simulink model "FSFB_FO_DoublePendulum"  (R2023b)
settings: Solver=VariableStepAuto  StartTime=0.0  StopTime=8  RelTol=1e-3
values from neighbouring files (symbols this model uses):
  A = [0 1 0 0; 9.8 0 -9.8 0; 0 0 0 1; -9.8 0 2.94 0]    [FSFB_FO_MIMO_doublePendulum.m]    (also in FSFB_MIMO_doublePendulum.m; FSFB_MO_MIMO_doublePendulum.m)
  B = [0 0; 1 -2; 0 0; -2 5]    [FSFB_FO_MIMO_doublePendulum.m]    (also in FSFB_MIMO_doublePendulum.m; FSFB_MO_MIMO_doublePendulum.m)
  C = [1 0 0 0; 0 0 1 0]    [FSFB_FO_MIMO_doublePendulum.m]    (also in FSFB_MIMO_doublePendulum.m; FSFB_MO_MIMO_doublePendulum.m)
  C_full = eye(max(size(A)))    [FSFB_FO_MIMO_doublePendulum.m]    (also in FSFB_MO_MIMO_doublePendulum.m)
  K_moore = W_moore/V_moore    [FSFB_FO_MIMO_doublePendulum.m]    (also in FSFB_MIMO_doublePendulum.m; FSFB_MO_MIMO_doublePendulum.m)
  L_moore = Q_moore\T    [FSFB_FO_MIMO_doublePendulum.m]
  L_moore_mr = Q_moore_mr\T    [FSFB_FO_MIMO_doublePendulum.m]
  x0 = [0 1 0 1]    [FSFB_FO_MIMO_doublePendulum.m]    (also in FSFB_MIMO_doublePendulum.m; FSFB_MO_MIMO_doublePendulum.m)
settings Model: Creator=frede  LastModifiedBy=frede

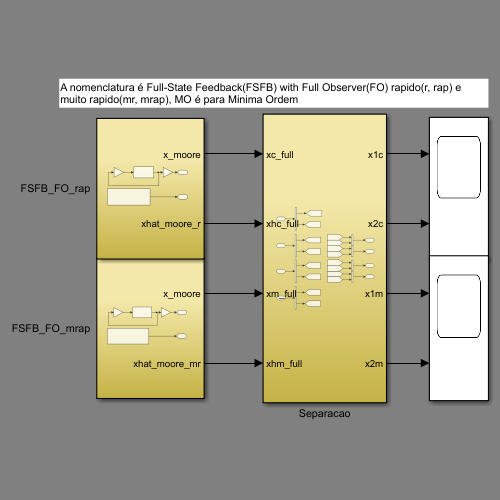
[thumbnail: Simulink's stored preview of the top-level diagram]
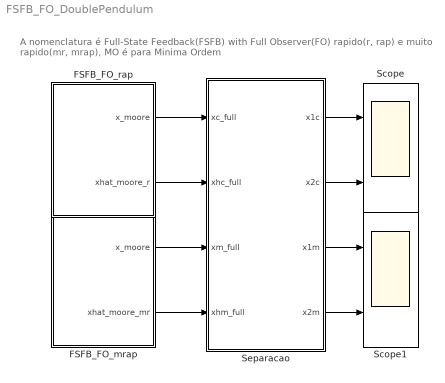
== system FSFB_FO_DoublePendulum ==
  note: A nomenclatura é Full-State Feedback(FSFB) with Full Observer(FO) rapido(r, rap) e muito rapido(mr, mrap), MO é para Minima Ordem
  FSFB_FO_mrap : Subsystem
  FSFB_FO_rap : Subsystem
  Scope : Scope  NumInputPorts=2
  Scope1 : Scope  NumInputPorts=2
  Separacao : Subsystem
  wires:
  FSFB_FO_mrap/1(x_moore) -> Separacao/3(xm_full)
  FSFB_FO_mrap/2(xhat_moore_mr) -> Separacao/4(xhm_full)
  Separacao/1(x1c) -> Scope/1
  Separacao/2(x2c) -> Scope/2
  Separacao/3(x1m) -> Scope1/1
  Separacao/4(x2m) -> Scope1/2
  FSFB_FO_rap/1(x_moore) -> Separacao/1(xc_full)
  FSFB_FO_rap/2(xhat_moore_r) -> Separacao/2(xhc_full)

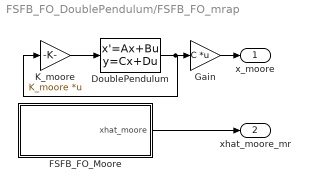
== system FSFB_FO_DoublePendulum/FSFB_FO_mrap ==
  DoublePendulum : StateSpace  A=A  B=B  C=eye(4)  D=zeros(4, 2)  InitialCondition=x0
  FSFB_FO_Moore : Subsystem
  Gain : Gain  Gain=C  Multiplication=Matrix(K*u)
  K_moore : Gain  Gain=K_moore  Multiplication=Matrix(K*u) (u vector)
  x_moore : Outport
  xhat_moore_mr : Outport  Port=2
  wires:
  K_moore/1 -> DoublePendulum/1
  DoublePendulum/1 -> K_moore/1, Gain/1
  FSFB_FO_Moore/1(xhat_moore) -> xhat_moore_mr/1
  Gain/1 -> x_moore/1

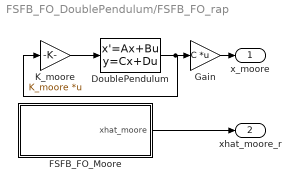
== system FSFB_FO_DoublePendulum/FSFB_FO_rap ==
  DoublePendulum : StateSpace  A=A  B=B  C=eye(4)  D=zeros(4, 2)  InitialCondition=x0
  FSFB_FO_Moore : Subsystem
  Gain : Gain  Gain=C  Multiplication=Matrix(K*u)
  K_moore : Gain  Gain=K_moore  Multiplication=Matrix(K*u) (u vector)
  x_moore : Outport
  xhat_moore_r : Outport  Port=2
  wires:
  K_moore/1 -> DoublePendulum/1
  DoublePendulum/1 -> K_moore/1, Gain/1
  FSFB_FO_Moore/1(xhat_moore) -> xhat_moore_r/1
  Gain/1 -> x_moore/1

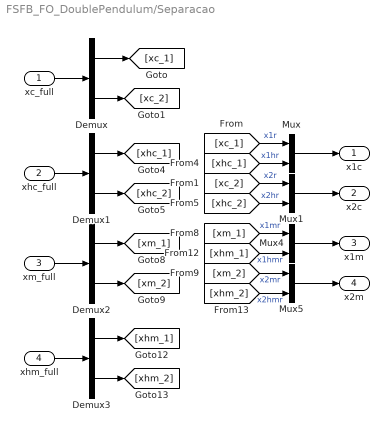
== system FSFB_FO_DoublePendulum/Separacao ==
  xc_full : Inport
  xhc_full : Inport  Port=2
  xm_full : Inport  Port=3
  xhm_full : Inport  Port=4
  Demux{,1..3} (4 alike) : Demux  Outputs=2
  Mux{,1,4..5} (4 alike) : Mux  Inputs=2
  x1c : Outport
  x2c : Outport  Port=2
  x1m : Outport  Port=3
  x2m : Outport  Port=4
  wires:
  [xhm_1] -> Mux4/2  "x1hmr"
  Demux/1 -> [xc_1]
  Demux3/1 -> [xhm_1]
  [xm_1] -> Mux4/1  "x1mr"
  Demux3/2 -> [xhm_2]
  [xc_1] -> Mux/1  "x1r"
  [xhm_2] -> Mux5/2  "x2hmr"
  Demux1/1 -> [xhc_1]
  [xc_2] -> Mux1/1  "x2r"
  [xhc_1] -> Mux/2  "x1hr"
  Demux2/1 -> [xm_1]
  Demux2/2 -> [xm_2]
  Mux1/1 -> x2c/1
  [xm_2] -> Mux5/1  "x2mr"
  xhm_full/1 -> Demux3/1
  Demux/2 -> [xc_2]
  [xhc_2] -> Mux1/2  "x2hr"
  Demux1/2 -> [xhc_2]
  Mux4/1 -> x1m/1
  Mux5/1 -> x2m/1
  xc_full/1 -> Demux/1
  xhc_full/1 -> Demux1/1
  xm_full/1 -> Demux2/1
  Mux/1 -> x1c/1

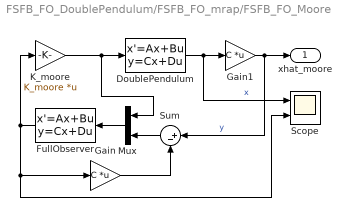
== system FSFB_FO_DoublePendulum/FSFB_FO_mrap/FSFB_FO_Moore ==
  "DoublePendulum  " : StateSpace  A=A  B=B  C=eye(4)  D=zeros(4, 2)  InitialCondition=x0
  FullObserver : StateSpace  A=A  B=[B L_moore_mr]  C=C_full  D=zeros(4,4)  InitialCondition=0
  Gain : Gain  Gain=C  Multiplication=Matrix(K*u) (u vector)
  Gain1 : Gain  Gain=C  Multiplication=Matrix(K*u) (u vector)
  K_moore : Gain  Gain=K_moore  Multiplication=Matrix(K*u) (u vector)
  Mux : Mux  Inputs=2
  Scope : Scope  NumInputPorts=2
  Sum : Sum  Inputs=|+-
  xhat_moore : Outport
  wires:
  "DoublePendulum  "/1 -> Gain1/1, Scope/1  "x"
  FullObserver/1 -> Scope/2, Gain/1, K_moore/1
  Mux/1 -> FullObserver/1
  Gain/1 -> Sum/2
  K_moore/1 -> Mux/1, "DoublePendulum  "/1
  Sum/1 -> Mux/2
  Gain1/1 -> xhat_moore/1, Sum/1  "y"

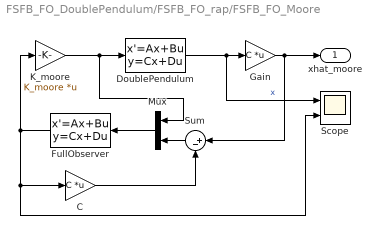
== system FSFB_FO_DoublePendulum/FSFB_FO_rap/FSFB_FO_Moore ==
  C : Gain  Gain=C  Multiplication=Matrix(K*u) (u vector)
  "DoublePendulum  " : StateSpace  A=A  B=B  C=eye(4)  D=zeros(4, 2)  InitialCondition=x0
  FullObserver : StateSpace  A=A  B=[B L_moore]  C=C_full  D=zeros(4,4)  InitialCondition=0
  Gain : Gain  Gain=C  Multiplication=Matrix(K*u) (u vector)
  K_moore : Gain  Gain=K_moore  Multiplication=Matrix(K*u) (u vector)
  Mux : Mux  Inputs=2
  Scope : Scope  NumInputPorts=2
  Sum : Sum  Inputs=|+-
  xhat_moore : Outport
  wires:
  "DoublePendulum  "/1 -> Scope/1, Gain/1  "x"
  FullObserver/1 -> C/1, Scope/2, K_moore/1
  K_moore/1 -> Mux/1, "DoublePendulum  "/1
  Mux/1 -> FullObserver/1
  C/1 -> Sum/2
  Sum/1 -> Mux/2
  Gain/1 -> Sum/1, xhat_moore/1
